simulink model "Clth_DD"  (R2016b)
settings: configuration reference "CodeGenConfigSet" (kept outside this file)
values from neighbouring files (symbols this model uses):
  Clth_stDflVal_C = Calibration.Parameter    [init_Clth_DD.m]
  Clth_swtSig_C = Calibration.Parameter    [init_Clth_DD.m]
  Clth_tiDebHiLo_C = Calibration.Parameter    [init_Clth_DD.m]
  Clth_tiDebLoHi_C = Calibration.Parameter    [init_Clth_DD.m]
  SigTst_stClth_C = Calibration.Parameter    [init_Clth_DD.m]
  SigTst_swtClth_C = Calibration.Parameter    [init_Clth_DD.m]
undefined symbols (not defined in the file or in its folder): Clth_DD_DT, Switch_conv
libraries: simulink x2, CXLib x1
settings Model: Creator=lenovo  LastModifiedBy=lenovo
settings ConfigSetRef: SourceLocation=Base Workspace

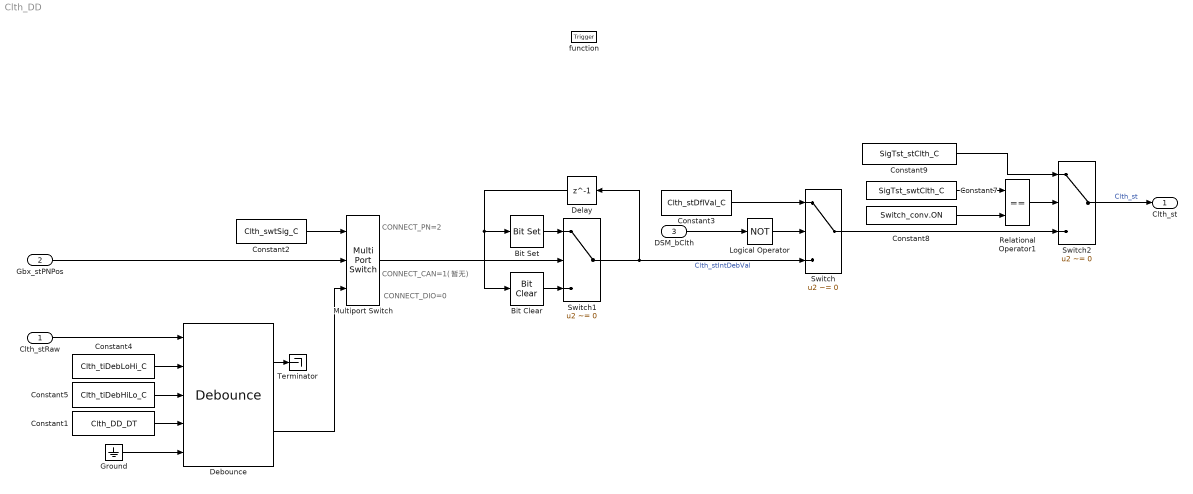
== system Clth_DD ==
  note: CONNECT_PN=2
  note: CONNECT_CAN=1(暂无)
  note: CONNECT_DIO=0
  Clth_stRaw : Inport  Description=Raw signal of clutch state  OutMin=0  OutMax=255  OutDataTypeStr=State_uint8
  Gbx_stPNPos : Inport  Description=Park Neutral Switch status  Port=2  OutMin=0  OutMax=255  OutDataTypeStr=State_uint8
  DSM_bClth : Inport  Description=state of Fid_Clth  Port=3  OutMin=0  OutMax=1  OutDataTypeStr=boolean
  function : TriggerPort  TriggerType=function-call  VariantControl=Variant
  Bit Clear : simulink/Logic and Bit Operations/Bit Clear  iBit=0
  Bit Set : simulink/Logic and Bit Operations/Bit Set  iBit=0
  Constant1 : Constant  Value=Clth_DD_DT  VectorParams1D=off  OutDataTypeStr=Inherit: Inherit via back propagation
  Constant2 : Constant  RequirementInfo={'other' 'Clth_requirements.doc' '@Simulink_requirement_item_2' 'true' '对离合器输入信号进行选择' '' } %GIDa_eba98797_aa5d_4d71_8b96_8811d64ef59d  Value=Clth_swtSig_C
  Constant3 : Constant  RequirementInfo={'other' 'Clth_requirements.doc' '@Simulink_requirement_item_3' 'true' '当离合器功能使能标志禁止时，输出默认状态' '' } %GIDa_9948d3b5_762c_4def_a2f2_69dc4ce25e80  Value=Clth_stDflVal_C
  Constant4 : Constant  Value=Clth_tiDebLoHi_C
  Constant5 : Constant  Value=Clth_tiDebHiLo_C  VectorParams1D=off
  Constant7 : Constant  Value=SigTst_swtClth_C
  Constant8 : Constant  Value=Switch_conv.ON
  Constant9 : Constant  Value=SigTst_stClth_C
  Debounce : CXLib/Debounce  RequirementInfo={'other' 'Clth_requirements.doc' '@Simulink_requirement_item_1' 'true' '对输入的离合器信号进行去抖处理，防止信号抖动' '' } %GIDa_73a273d4_6947_4a69_844d_15f805442b5e
  Delay : Delay  DelayLength=1  InitialCondition=0
  Ground : Ground
  Logical Operator : Logic  Operator=NOT  AllPortsSameDT=off  OutDataTypeStr=boolean
  Multiport Switch : MultiPortSwitch  RequirementInfo={'other' 'Clth_requirements.doc' '@Simulink_requirement_item_2' 'true' '对离合器输入信号进行选择' '' } %GIDa_88b80908_eff1_448c_bf96_650bba9e897d  DataPortOrder=Specify indices  DataPortIndices={2,0}
  Relational Operator1 : RelationalOperator  Operator===  OutDataTypeStr=boolean  RndMeth=Nearest
  Switch : Switch  RequirementInfo={'other' 'Clth_requirements.doc' '@Simulink_requirement_item_3' 'true' '当离合器功能使能标志禁止时，输出默认状态' '' } %GIDa_788e42e0_fc1f_4cba_94a4_c8b5079b0a46  Criteria=u2 ~= 0  OutDataTypeStr=Inherit: Inherit via back propagation  InputSameDT=on
  Switch1 : Switch  Criteria=u2 ~= 0  OutDataTypeStr=Inherit: Inherit via back propagation  InputSameDT=on
  Switch2 : Switch  RequirementInfo={'other' 'Clth_requirements.doc' '@Simulink_requirement_item_3' 'true' '当离合器功能使能标志禁止时，输出默认状态' '' } %GIDa_2b60a46a_3460_484a_bf2d_a04c05515137  Criteria=u2 ~= 0  OutDataTypeStr=Inherit: Inherit via back propagation  InputSameDT=on
  Terminator : Terminator
  Clth_st : Outport  Description=Clutch information  OutMin=0  OutMax=255  OutDataTypeStr=State_uint8
  wires:
  Constant3/1 -> Switch/1
  Switch2/1 -> Clth_st/1  "Clth_st"
  Constant9/1 -> Switch2/1
  Relational Operator1/1 -> Switch2/2
  Constant7/1 -> Relational Operator1/1
  Constant8/1 -> Relational Operator1/2
  Switch/1 -> Switch2/3
  Multiport Switch/1 -> Switch1/2
  Gbx_stPNPos/1 -> Multiport Switch/2
  Delay/1 -> Bit Set/1, Bit Clear/1
  Bit Clear/1 -> Switch1/3
  Bit Set/1 -> Switch1/1
  Switch1/1 -> Delay/1, Switch/3  "Clth_stIntDebVal"
  Logical Operator/1 -> Switch/2
  DSM_bClth/1 -> Logical Operator/1
  Debounce/2 -> Multiport Switch/3
  Debounce/1 -> Terminator/1
  Ground/1 -> Debounce/5
  Constant1/1 -> Debounce/4
  Constant5/1 -> Debounce/3
  Constant4/1 -> Debounce/2
  Clth_stRaw/1 -> Debounce/1
  Constant2/1 -> Multiport Switch/1
